simulink model "trigger_fromfile"  (R2013a)
settings: Solver=VariableStepDiscrete  StartTime=0.0  StopTime=15  RelTol=1e-3
InitFcn:
  | fs_file=20e3;
  | decLpfB=[8.576557e-06, 5.145934e-05, 1.286484e-04, 1.715311e-04, 1.286484e-04, 5.145934e-05, 8.576557e-06, ];
  | decLpfA=[1.000000e+00, -4.787135e+00, 9.649518e+00, -1.046908e+01, 6.441112e+00, -2.129039e+00, 2.951724e-01, ];
  | decimationFactor=10;
  | lpfB=[2.433749e-03, 4.723405e-03, 8.336385e-03, 9.237523e-03, 8.336385e-03, 4.723405e-03, 2.433749e-03, ];
  | lpfA=[1.000000e+00, -3.892269e+00, 7.296388e+00, -8.110266e+00, 5.586567e+00, -2.254573e+00, 4.192858e-01, ];
  | windowSize=1000;
  | alpha=2e-6;
libraries: dspsigops x1, simulink x1
settings Model: Creator=balazs.varga  LastModifiedBy=balazs.varga

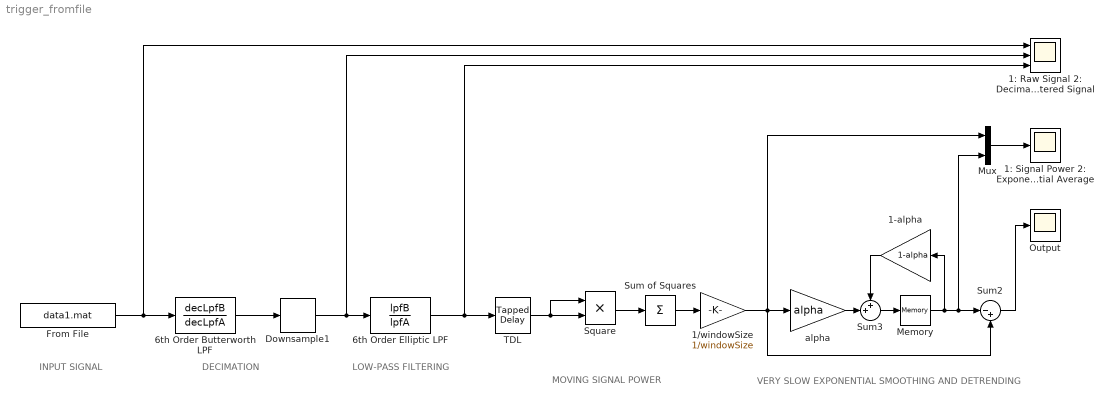
== system trigger_fromfile ==
  note: VERY SLOW EXPONENTIAL SMOOTHING
      | AND DETRENDING
  note: MOVING SIGNAL POWER
  note: INPUT SIGNAL
  note: LOW-PASS FILTERING
  note: DECIMATION
  1-alpha : Gain  Gain=1-alpha  SampleTime=1/(fs_file/decimationFactor)
  1/windowSize : Gain  Gain=1/windowSize  SampleTime=1/(fs_file/decimationFactor)
  1: Raw Signal 2: Decimated Signal 3: Filtered Signal : Scope  NumInputPorts=3
      settings: YMin=-5~-5~-5  YMax=5~5~5
  1: Signal Power 2: Exponential Average : Scope
      settings: YMin=0  YMax=525  SaveName=ScopeData3
  6th Order Butterworth LPF : DiscreteFilter  Numerator=decLpfB  Denominator=decLpfA  SampleTime=1/fs_file
  6th Order Elliptic LPF : DiscreteFilter  Numerator=lpfB  Denominator=lpfA  SampleTime=1/(fs_file/decimationFactor)
  Downsample1 : dspsigops/Downsample  N=decimationFactor  phase=0  InputProcessing=Columns as channels (frame based)  RateOptions=Allow multirate processing  smode=Allow multirate  fmode=Maintain input frame size  ic=0
  From File : FromFile  FileName=data1.mat  SampleTime=1/fs_file
  Memory : Memory  InheritSampleTime=on
  Mux : Mux  Inputs=2
  Output : Scope
      settings: YMin=-0.1  YMax=2.2  SaveName=ScopeData2
  Square : Product  SampleTime=1/(fs_file/decimationFactor)
  Sum of Squares : Sum  Inputs=+  SampleTime=1/(fs_file/decimationFactor)
  Sum2 : Sum  Inputs=|-+  SampleTime=1/(fs_file/decimationFactor)
  Sum3 : Sum  Inputs=++|  SampleTime=1/(fs_file/decimationFactor)
  TDL : simulink/Discrete/Tapped Delay  vinit=0.0  samptime=1/(fs_file/decimationFactor)  NumDelays=windowSize-1  DelayOrder=Newest  includeCurrent=on
  alpha : Gain  Gain=alpha  SampleTime=1/(fs_file/decimationFactor)
  wires:
  6th Order Elliptic LPF/1 -> 1: Raw Signal 2: Decimated Signal 3: Filtered Signal/3, TDL/1
  TDL/1 -> Square/2, Square/1
  Square/1 -> Sum of Squares/1
  Sum3/1 -> Memory/1
  alpha/1 -> Sum3/2
  1-alpha/1 -> Sum3/1
  Memory/1 -> 1-alpha/1, Sum2/1, Mux/2
  Mux/1 -> 1: Signal Power 2: Exponential Average/1
  Sum of Squares/1 -> 1/windowSize/1
  Sum2/1 -> Output/1
  1/windowSize/1 -> alpha/1, Sum2/2, Mux/1
  From File/1 -> 1: Raw Signal 2: Decimated Signal 3: Filtered Signal/1, 6th Order Butterworth LPF/1
  Downsample1/1 -> 1: Raw Signal 2: Decimated Signal 3: Filtered Signal/2, 6th Order Elliptic LPF/1
  6th Order Butterworth LPF/1 -> Downsample1/1
